simulink model "SimulationStateFeedbackController_ObserverBased"  (Simulink 7.8)
settings: Solver=ode1  StartTime=0.0  StopTime=30  FixedStep=T  RelTol=1e-3
values from neighbouring files (symbols this model uses):
  A = [zero I;-inv(M_bar)*K_bar zero]    [ABC.m]    (also in Lab1Demo_Sys.m = [0              1               0               0)
  B = [zero;inv(M_bar)]*[1;0]    [ABC.m]    (also in Lab1Demo_Sys.m = [0 0 0 1/m2]')
  C = [1 0 0 0;0 1 0 0]    [ABC.m]
  K = place(A,B,DesK)    [ABC.m]
  L = Lt'    [ABC.m]
  T = 0.001    [ABC.m]    (also in lab_param.m)
  X0 = [pi/2+.1 -.05 0 0]    [ABC.m]    (also in Constants.m = [pi/2 -pi 0 0]'; Lab1DemoParam.m = [.05 0 -.02 0])
undefined symbols (not defined in the file or in its folder): DiscIntNeverNeededParam, Parameters
settings Model: Creator=jafarm2  LastModifiedBy=jafarm2  ExtModeTrigDuration=5000
settings SolverCC: PositivePriorityOrder=on
settings RTWCC: SystemTargetFile=quarc_win64.tlc  TemplateMakefile=quarc_default_tmf  Description=QUARC Win64 Target  ProcessScript=quarc_win64_make_rtw_hook
settings STFCustomTargetCC: TargetPreCompLibLocation=C:\PROGRA~3\QUARC\lib\2011b\win64\release  SystemTargetFile=quarc_win64.tlc
settings GRTTargetCC: TargetPreCompLibLocation=C:\PROGRA~3\QUARC\lib\2011b\win64\release  ParMdlRefBuildCompliant=off  CompOptLevelCompliant=off  ConcurrentExecutionCompliant=off  MatFileLogging=off  ExtMode=on  ExtModeMexFile=quarc_comm

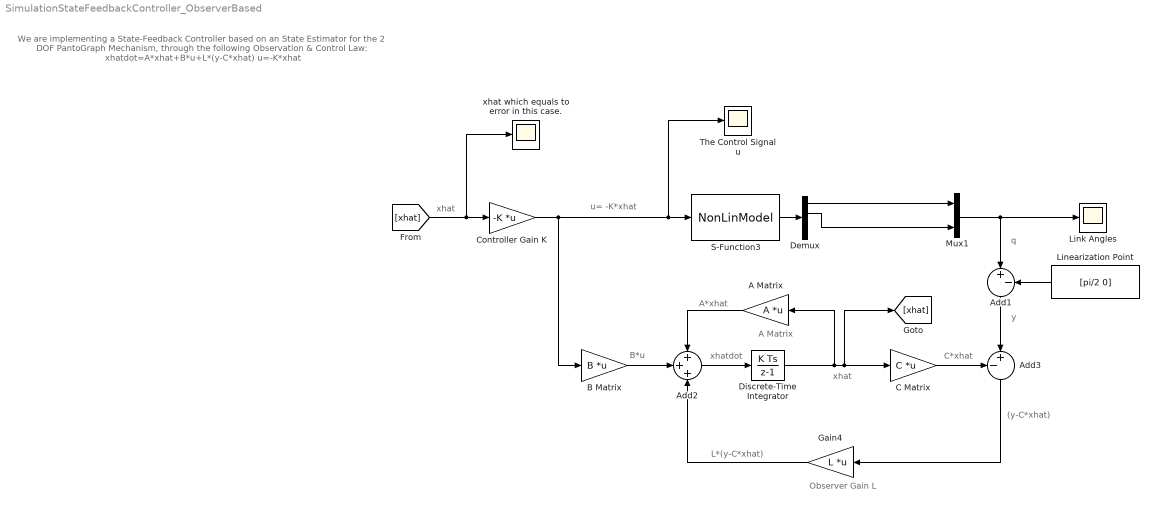
== system SimulationStateFeedbackController_ObserverBased ==
  note: q
  note: y
  note: B*u
  note: A Matrix
  note: A*xhat
  note: xhat
  note: C*xhat
  note: (y-C*xhat)
  note: L*(y-C*xhat)
  note: Observer Gain L
  note: u= -K*xhat
  note: xhat
  note: xhatdot
  note: We are implementing a State-Feedback Controller based on an State Estimator for the 2 DOF PantoGraph Mechanism,
      | through the following Observation & Control Law:
      | xhatdot=A*xhat+B*u+L*(y-C*xhat)
      | u=-K*xhat
  A Matrix : Gain  Gain=A  Multiplication=Matrix(K*u)
  Add1 : Sum  Inputs=|+-
  Add2 : Sum  Inputs=+++
  Add3 : Sum  Inputs=-+|
  B Matrix : Gain  Gain=B  Multiplication=Matrix(K*u)
  C Matrix : Gain  Gain=C  Multiplication=Matrix(K*u)
  Controller Gain K : Gain  Gain=-K  Multiplication=Matrix(K*u)
  Demux : Demux
  Discrete-Time Integrator : DiscreteIntegrator  InitialCondition=[0 0 0 0]'  SampleTime=T  ICPrevOutput=DiscIntNeverNeededParam  ICPrevScaledInput=DiscIntNeverNeededParam
  Gain4 : Gain  Gain=L  Multiplication=Matrix(K*u)
  Linearization Point : Constant  Value=[pi/2 0]
  Link Angles : Scope
      settings: YMin=-0.25  YMax=1.75
  Mux1 : Mux  Inputs=2
  S-Function3 : S-Function  FunctionName=NonLinModel  Parameters=X0,Parameters  EnableBusSupport=off
  The Control Signal u : Scope
      settings: TimeRange=20  YMin=-110  YMax=110  SaveName=ScopeData3
  xhat which equals to error in this case. : Scope
      settings: YMin=-0.00024  YMax=-0.0001
  wires:
  Controller Gain K/1 -> B Matrix/1, The Control Signal u/1, S-Function3/1
  Mux1/1 -> Link Angles/1, Add1/1
  Demux/1 -> Mux1/1
  Demux/2 -> Mux1/2
  Add2/1 -> Discrete-Time Integrator/1
  C Matrix/1 -> Add3/1
  Add3/1 -> Gain4/1
  Discrete-Time Integrator/1 -> A Matrix/1, C Matrix/1, [xhat]
  B Matrix/1 -> Add2/2
  A Matrix/1 -> Add2/1
  Add1/1 -> Add3/2
  Linearization Point/1 -> Add1/2
  Gain4/1 -> Add2/3
  [xhat] -> Controller Gain K/1, xhat which equals to error in this case./1
  S-Function3/1 -> Demux/1
